simulink model "Group3_HEV_model"  (Simulink 7.9)
settings: Solver=ode4  StartTime=0.0  StopTime=Stoptime  FixedStep=1  MaxStep=.05  RelTol=1e-3
InitFcn:
  | load Mat_files/ENV_Data.mat;
  | load Mat_files/TRAN_Data.mat;
  | load Mat_files/VEH_Data.mat;
  | load Mat_files/TC_Data.mat;
  | load Mat_files/Drive_cycle.mat;
  | load Mat_files/ICE_Data.mat;
  | load Mat_files/EM_Data.mat;
  | load Mat_files/BATT_Data.mat
  | clc;
  | %warning off all;
StopFcn:
  | disp('Simulation Complete.')
values from neighbouring files (symbols this model uses):
  EM = EM2    [Group3_Plot.m]
  EM2 =     [EM2_map.mat]
  em_trq_e_g1 = em_trq_e    [Group3_ECMS_control_strategy.m]    (also in ecms_table_n5.mat = [-2 -2 -2 -2 -2 -2 -2 -2 -2 -2 -2 -2 ... (715 elements, 11x1)
  em_trq_e_g2 = em_trq_e    [Group3_ECMS_control_strategy.m]    (also in ecms_table_n5.mat = [-2 -2 -2 -2 -2 -2 -2 -2 -2 -2 -2 -2 ... (715 elements, 11x1)
  em_trq_e_g3 = em_trq_e    [Group3_ECMS_control_strategy.m]    (also in ecms_table_n5.mat = [-2 -2 -2 -2 -2 -2 -2 -2 -2 -2 -2 -2 ... (715 elements, 11x1)
  fs_0 = 1    [Group3_Initialization.m]
  fs_act = 1    [Group3_Initialization.m]
  hA_0 = 0.07    [Group3_Initialization.m]
  ICE =     [Engine2_map.mat]
  ice_w_e = linspace(0,50*m2,m2+1)    [Group3_ECMS_control_strategy.m]    (also in ecms_table_n5.mat = [0 50 100 150 200 250 300 350 400 450 500])
  mc = 50    [Group3_Initialization.m]
  N = 250    [Group3_Initialization.m]
  soc_e = linspace(-1,1,m3)    [Group3_ECMS_control_strategy.m]    (also in ecms_table_n5.mat = [-1 -0.5 0 0.5 1])
  soc_h = 0.85    [Group3_ECMS_control_strategy.m]    (also in Group3_Initialization.m)
  soc_l = 0.55    [Group3_ECMS_control_strategy.m]    (also in Group3_Initialization.m)
  Sport = 1    [Group3_Initialization.m]
  T_amb = 20+273    (= 293)    [Group3_Initialization.m]
  Treq = linspace(0,20*m1,m1+1)    [Group3_ECMS_control_strategy.m]    (also in ecms_table_n5.mat = [0 20 40 60 80 100 120 140 160 180 200 220 ... (13 elements,)
undefined symbols (not defined in the file or in its folder): BATT, ENV, TC, TRAN, VEH
libraries: simulink x6
(part 2 of 2)

== system Group3_HEV_model/Hybrid-Electric Powertrain/CONTROLLER/Primary Control/Torque Controller/EM sort   propulsion/ regen ==
  EM_torque : Inport
  Constant{1..3,14} (4 alike) : Constant  Value=0
  SOC Limit (Motoring)2 : Switch  Criteria=u2 > Threshold  Threshold=.55
  SOC Limit (Regen)2 : Switch  Criteria=u2 > Threshold  Threshold=.85
  "propulsion " : Switch
  regen : Switch
  Torque _power : Outport
  Torque_regene : Outport  Port=2
  wires:
  [BATT_SOC] -> SOC Limit (Motoring)2/2
  Constant14/1 -> SOC Limit (Motoring)2/3
  EM_torque/1 -> "propulsion "/2, regen/2, regen/3, "propulsion "/1
  regen/1 -> SOC Limit (Regen)2/3
  Constant1/1 -> regen/1
  Constant2/1 -> "propulsion "/3
  "propulsion "/1 -> SOC Limit (Motoring)2/1
  Constant3/1 -> SOC Limit (Regen)2/1
  [BATT_SOC] -> SOC Limit (Regen)2/2
  SOC Limit (Regen)2/1 -> Torque_regene/1
  SOC Limit (Motoring)2/1 -> Torque _power/1

== system Group3_HEV_model/Hybrid-Electric Powertrain/CONTROLLER/Primary Control/Torque Controller/Prevent Drawing Too Much Power From The Battery1 ==
  In1 : Inport
  Constant1 : Constant  Value=0
  Constant2 : Constant  Value=.001
  Constant3 : Constant  Value=30000
  Divide : Product  Inputs=*/
  Memory3 : Memory
  Saturation Dynamic : simulink/Discontinuities/Saturation Dynamic  OutMin=[]  OutMax=[]  OutDataTypeStr=Inherit: Same as second input  OutDataType=sfix(16)  OutScaling=2^-10  DoSatur=off
  Switch : Switch  Criteria=u2 > Threshold
  Out2 : Outport
  wires:
  Constant1/1 -> Saturation Dynamic/3
  In1/1 -> Saturation Dynamic/2
  Saturation Dynamic/1 -> Out2/1
  Divide/1 -> Memory3/1
  Memory3/1 -> Saturation Dynamic/1
  [EM_w] -> Switch/2
  Switch/1 -> Divide/2
  Constant2/1 -> Switch/3
  [EM_w] -> Switch/1
  Constant3/1 -> Divide/1

== system Group3_HEV_model/Hybrid-Electric Powertrain/CONTROLLER/Primary Control/Torque Controller/Prevent Over-Charging  The Battery2 ==
  In1 : Inport
  Constant1 : Constant  Value=0
  Constant2 : Constant  Value=.001
  Constant3 : Constant  Value=-30000
  Divide : Product  Inputs=*/
  Memory3 : Memory
  Saturation Dynamic : simulink/Discontinuities/Saturation Dynamic  OutMin=[]  OutMax=[]  OutDataTypeStr=Inherit: Same as second input  OutDataType=sfix(16)  OutScaling=2^-10  DoSatur=off
  Switch : Switch  Criteria=u2 > Threshold
  Out2 : Outport
  wires:
  In1/1 -> Saturation Dynamic/2
  Saturation Dynamic/1 -> Out2/1
  Divide/1 -> Memory3/1
  [EM_w] -> Switch/2
  Switch/1 -> Divide/2
  Constant2/1 -> Switch/3
  [EM_w] -> Switch/1
  Constant1/1 -> Saturation Dynamic/1
  Memory3/1 -> Saturation Dynamic/3
  Constant3/1 -> Divide/1

== system Group3_HEV_model/Hybrid-Electric Powertrain/CONTROLLER/Primary Control/Torque Controller/Subsystem ==
  T_req : Inport
  ice_w : Inport  Port=2
  battery_soc : Inport  Port=3
  trans gear : Inport  Port=4
  Merge : Merge  Inputs=4
  Mux : Mux  Inputs=3
  Switch Case Action Subsystem : Subsystem  TreatAsAtomicUnit=on
  Switch Case Action Subsystem1 : Subsystem  TreatAsAtomicUnit=on
  Switch Case Action Subsystem2 : Subsystem  TreatAsAtomicUnit=on
  Switch Case Action Subsystem4 : Subsystem  TreatAsAtomicUnit=on
  Switch Case1 : SwitchCase  CaseConditions={1,2,3}
  Out1 : Outport
  wires:
  T_req/1 -> Mux/1
  ice_w/1 -> Mux/2
  battery_soc/1 -> Mux/3
  trans gear/1 -> Switch Case1/1
  Switch Case1/1 -> Switch Case Action Subsystem/Action
  Mux/1 -> Switch Case Action Subsystem2/1(In1), Switch Case Action Subsystem4/1(In1), Switch Case Action Subsystem1/1(In1), Switch Case Action Subsystem/1(In1)
  Switch Case1/2 -> Switch Case Action Subsystem1/Action
  Switch Case1/3 -> Switch Case Action Subsystem2/Action
  Switch Case Action Subsystem/1(Out1) -> Merge/1
  Switch Case Action Subsystem1/1(Out1) -> Merge/2
  Switch Case Action Subsystem2/1(Out1) -> Merge/3
  Switch Case Action Subsystem4/1(Out1) -> Merge/4
  Merge/1 -> Out1/1
  Switch Case1/4 -> Switch Case Action Subsystem4/Action

== system Group3_HEV_model/Hybrid-Electric Powertrain/CONTROLLER/Primary Control/Torque Controller/breaking ==
  In1 : Inport
  Constant12 : Constant  Value=0
  Constant20 : Constant  Value=EM2.maxT_T
  Gain1 : Gain  Gain=-1
  MinMax5 : MinMax  Function=max
  Product5 : Product  RndMeth=Zero
  SOC Limit (Regen)1 : Switch  Criteria=u2 > Threshold  Threshold=.85
  Out1 : Outport
  wires:
  Constant20/1 -> MinMax5/1
  MinMax5/1 -> Gain1/1
  Gain1/1 -> Product5/2
  SOC Limit (Regen)1/1 -> Out1/1
  [BATT_SOC] -> SOC Limit (Regen)1/2
  Constant12/1 -> SOC Limit (Regen)1/1
  Product5/1 -> SOC Limit (Regen)1/3
  In1/1 -> Product5/1

== system Group3_HEV_model/Hybrid-Electric Powertrain/CONTROLLER/Primary Control/Torque Controller/torque request ==
  In1 : Inport
  Product3 : Product  RndMeth=Zero
  max torqe request : Constant  Value=510
  Out1 : Outport
  wires:
  max torqe request/1 -> Product3/2
  In1/1 -> Product3/1
  Product3/1 -> Out1/1

== system Group3_HEV_model/Hybrid-Electric Powertrain/CONTROLLER/Primary Control/Torque Controller/x_soc ==
  In1 : Inport
  Aerodynamic Force1 : ToWorkspace  VariableName=x_soc  SampleTime=-1
  Saturation1 : Saturate
  x_soc1 : Fcn  Expr=(u^1-(soc_h+soc_l)/2)/((soc_h-soc_l)/2)
  Out1 : Outport
  wires:
  In1/1 -> x_soc1/1
  x_soc1/1 -> Saturation1/1, Aerodynamic Force1/1
  Saturation1/1 -> Out1/1

== system Group3_HEV_model/Hybrid-Electric Powertrain/High-Voltage Battery & Switch Box2/R Circuit/THERMAL MODEL/Fan setting = 0 ==
  Action Port : ActionPort  ActionType=else
  Fan setting : Constant  Value=0
  fs0 : Outport
  wires:
  Fan setting/1 -> fs0/1

== system Group3_HEV_model/Hybrid-Electric Powertrain/High-Voltage Battery & Switch Box2/R Circuit/THERMAL MODEL/Fan setting = 1 ==
  Action Port : ActionPort  ActionType=elseif
  Fan setting : Constant
  fs1 : Outport
  wires:
  Fan setting/1 -> fs1/1

== system Group3_HEV_model/Hybrid-Electric Powertrain/High-Voltage Battery & Switch Box2/R Circuit/THERMAL MODEL/Fan setting = 2 ==
  Action Port : ActionPort  ActionType=elseif
  Fan setting : Constant  Value=2
  fs2 : Outport
  wires:
  Fan setting/1 -> fs2/1

== system Group3_HEV_model/Hybrid-Electric Powertrain/High-Voltage Battery & Switch Box2/R Circuit/THERMAL MODEL/Fan setting = 3 ==
  Action Port : ActionPort  ActionType=then
  Fan setting : Constant  Value=3
  fs3 : Outport
  wires:
  Fan setting/1 -> fs3/1

== system Group3_HEV_model/Hybrid-Electric Powertrain/CONTROLLER/Primary Control/Torque Controller/Subsystem/Switch Case Action Subsystem ==
  In1 : Inport
  Action Port : ActionPort  ActionType=case
  Demux : Demux  Outputs=3
  n-D Lookup Table : Lookup_n-D  NumberOfTableDimensions=3  BreakpointsForDimension1=ice_w_e  BreakpointsForDimension2=Treq  BreakpointsForDimension3=soc_e  Table=em_trq_e_g1  RndMeth=Simplest  InputSameDT=on
  Out1 : Outport
  wires:
  Demux/2 -> n-D Lookup Table/2
  Demux/1 -> n-D Lookup Table/1
  Demux/3 -> n-D Lookup Table/3
  In1/1 -> Demux/1
  n-D Lookup Table/1 -> Out1/1

== system Group3_HEV_model/Hybrid-Electric Powertrain/CONTROLLER/Primary Control/Torque Controller/Subsystem/Switch Case Action Subsystem1 ==
  In1 : Inport
  Action Port : ActionPort  ActionType=case
  Demux : Demux  Outputs=3
  n-D Lookup Table : Lookup_n-D  NumberOfTableDimensions=3  BreakpointsForDimension1=ice_w_e  BreakpointsForDimension2=Treq  BreakpointsForDimension3=soc_e  Table=em_trq_e_g2  RndMeth=Simplest  InputSameDT=on
  Out1 : Outport
  wires:
  Demux/2 -> n-D Lookup Table/2
  Demux/1 -> n-D Lookup Table/1
  Demux/3 -> n-D Lookup Table/3
  In1/1 -> Demux/1
  n-D Lookup Table/1 -> Out1/1

== system Group3_HEV_model/Hybrid-Electric Powertrain/CONTROLLER/Primary Control/Torque Controller/Subsystem/Switch Case Action Subsystem2 ==
  In1 : Inport
  Action Port : ActionPort  ActionType=case
  Demux : Demux  Outputs=3
  n-D Lookup Table : Lookup_n-D  NumberOfTableDimensions=3  BreakpointsForDimension1=ice_w_e  BreakpointsForDimension2=Treq  BreakpointsForDimension3=soc_e  Table=em_trq_e_g3  RndMeth=Simplest  InputSameDT=on
  Out1 : Outport
  wires:
  Demux/2 -> n-D Lookup Table/2
  Demux/1 -> n-D Lookup Table/1
  Demux/3 -> n-D Lookup Table/3
  In1/1 -> Demux/1
  n-D Lookup Table/1 -> Out1/1

== system Group3_HEV_model/Hybrid-Electric Powertrain/CONTROLLER/Primary Control/Torque Controller/Subsystem/Switch Case Action Subsystem4 ==
  In1 : Inport
  Action Port : ActionPort  ActionType=default
  Demux : Demux  Outputs=3
  n-D Lookup Table : Lookup_n-D  NumberOfTableDimensions=3  BreakpointsForDimension1=ice_w_e  BreakpointsForDimension2=Treq  BreakpointsForDimension3=soc_e  Table=em_trq_e_g1  RndMeth=Simplest  InputSameDT=on
  Out1 : Outport
  wires:
  Demux/2 -> n-D Lookup Table/2
  Demux/1 -> n-D Lookup Table/1
  Demux/3 -> n-D Lookup Table/3
  In1/1 -> Demux/1
  n-D Lookup Table/1 -> Out1/1
